simulink model "stage4"  (Simulink 7.7)
settings: Solver=ode45  StartTime=0.0  StopTime=0.1  RelTol=1e-3
undefined symbols (not defined in the file): Acid, Lead
libraries: powerlib x7, electricdrivelib x2
settings Model: Creator=Vikas  LastModifiedBy=HASANTH

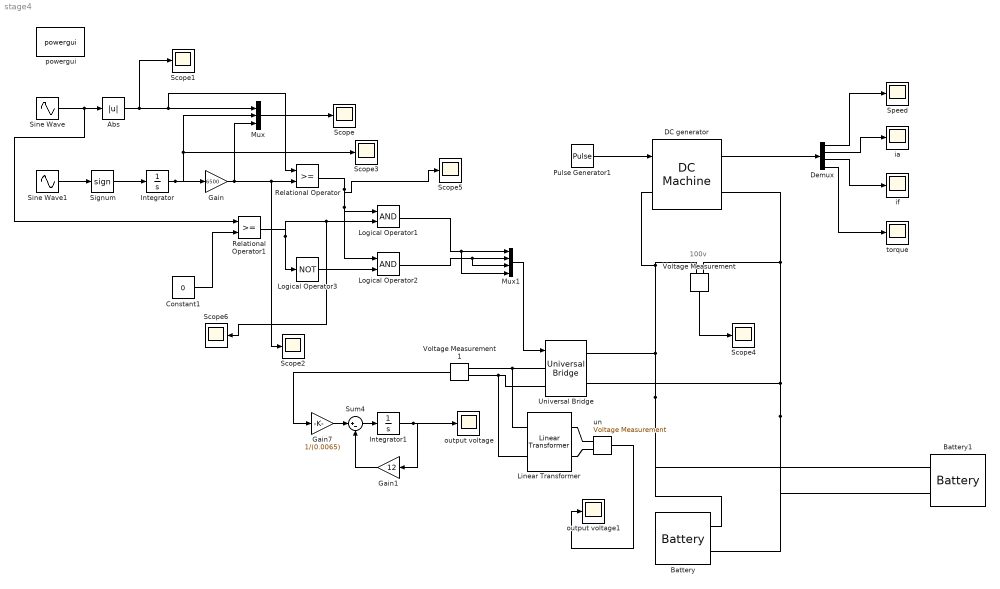
== system stage4 ==
  note: 100v
  Abs : Abs
  Battery : electricdrivelib/Extra Sources/Battery  SystemSampleTime=-1  BatType=Lead-Acid  ShowDetailedParameters=off  NomV=15  NomQ=60  SOC=20  PresetModel=on  MaxQ=62.5  FullV=16.3322  Dis_rate=12  R=0.0025  Normal_OP=18.6167  expZone="[15.2714          0.2]"  Dis_Char=off  current=[6.5 13 32.5]  Units=Time  Batt_Tr=5
  Battery1 : electricdrivelib/Extra Sources/Battery  SystemSampleTime=-1  BatType=Lead-Acid  ShowDetailedParameters=off  NomV=15  NomQ=60  SOC=20  PresetModel=on  MaxQ=62.5  FullV=16.3322  Dis_rate=12  R=0.0025  Normal_OP=18.6167  expZone="[15.2714          0.2]"  Dis_Char=off  current=[6.5 13 32.5]  Units=Time  Batt_Tr=5
  Constant1 : Constant  Value=0
  DC generator : powerlib/Machines/DC Machine  SystemSampleTime=-1  PresetModel=No  MechanicalLoad=Speed w  FieldType=Permanent magnet  ShowDetailedParameters=on  RLa="[ 1  0.012]"  RLf="[ 240  120]"  Laf=1.8  MachineConstant=Back-emf constant (V/rpm)  Ke=3  Kt=3.18  J=1  Bm=0  Tf=0  w0=1  Ifinit=1  TsPowergui=0  TsBlock=-1
      settings: AttributesFormatString=\n
  Demux : Demux
  Gain : Gain  Gain=6500
  Gain1 : Gain  Gain=12
  Gain7 : Gain  Gain=1/(0.0065)
  Integrator : Integrator
  Integrator1 : Integrator
  Linear Transformer : powerlib/Elements/Linear Transformer  PhysicalDomain=powersysdomain  SubClassName=unknown  LeftPortType=p1  RightPortType=p1  LConnTagsString=a|b  RConnTagsString=A|B  UNITS=pu  NominalPower=[ 875 50 ]  winding1="[15  0.002  0.08 ]"  winding2="[240  0.002  0.08 ]"  ThreeWindings=off  winding3=[ 315e3 0.002 0.08 ]  RmLm=[ 500 500 ]  Measurements=None  DataType=off
  Logical Operator1 : Logic  AllPortsSameDT=off  OutDataTypeStr=boolean
  Logical Operator2 : Logic  AllPortsSameDT=off  OutDataTypeStr=boolean
  Logical Operator3 : Logic  Operator=NOT  AllPortsSameDT=off  OutDataTypeStr=boolean
  Mux : Mux  Inputs=3
  Mux1 : Mux
  Pulse Generator1 : DiscretePulseGenerator  PulseType=Time based  Amplitude=5.4  Period=10  PulseWidth=50
  Relational Operator : RelationalOperator  InputSameDT=on
  Relational Operator1 : RelationalOperator  InputSameDT=on
  Scope{,1..6} (7 alike) : Scope
      Scope settings: TimeRange=10  YMin=-0.1  YMax=2.1  SaveName=ScopeData5
      Scope1 settings: TimeRange=10  YMin=-0.1  YMax=2.1  SaveName=ScopeData8
      Scope2 settings: TimeRange=10  YMin=-0.1  YMax=2.1  SaveName=ScopeData6
      Scope3 settings: TimeRange=10  YMin=-0.1  YMax=2.1  SaveName=ScopeData7
      Scope4 settings: TimeRange=1  YMin=0  YMax=36.0525  SaveName=ScopeData4
      Scope5 settings: TimeRange=10  YMin=-0.1  YMax=2.1  SaveName=ScopeData9
      Scope6 settings: TimeRange=10  YMin=-0.1  YMax=2.1  SaveName=ScopeData11
  Signum : Signum
  Sine Wave : Sin  Frequency=2*pi*50  SampleTime=0
  Sine Wave1 : Sin  Frequency=2*pi*3000  SampleTime=0
  Speed : Scope
  Sum4 : Sum  Inputs=|+-
  Universal Bridge : powerlib/Power Electronics/Universal Bridge  SystemSampleTime=-1  Arms=2  SnubberResistance=1e5  SnubberCapacitance=inf  Device=MOSFET / Diodes  Ron=1e-3  Lon=0  ForwardVoltages="[  0  0  ]"  ForwardVoltage=0  GTOparameters=[ 10e-6 , 20e-6 ]  IGBTparameters=[ 1e-6 , 2e-6 ]  Measurements=None  Measurements_2=None  converterType=Rectifier
  Voltage Measurement : powerlib/Measurements/Voltage Measurement  SystemSampleTime=-1  PhasorSimulation=off  OutputType=Complex  PSBequivalent=0
  Voltage Measurement1 : powerlib/Measurements/Voltage Measurement  SystemSampleTime=-1  PhasorSimulation=off  OutputType=Complex  PSBequivalent=0
  ia : Scope
  if : Scope
      settings: SaveName=ScopeData2
  output voltage : Scope
      settings: YMin=0.3523  YMax=0.3538  SaveName=ScopeData10
  output voltage1 : Scope
      settings: YMin=4.5e-010  YMax=7.75e-010  SaveName=ScopeData12
  powergui : powerlib/powergui  Priority=1  SystemSampleTime=-1  SimulationMode=Continuous  SampleTime=50e-6  frequency=60  SPID=off  DisableSnubberDevices=off  DisableRonSwitches=off  DisableVfSwitches=off  SwTol=0  Interpol=off  DisplayEquations=off  FunctionMessages=off  frequencyindice=0  Pbase=100e6  ErrMax=1e-4  Iterations=50  UnitsV=kV  UnitsW=MW  echomessages=off  HookPort=off  EnableUseOfTLC=off  x0status=steady  RestoreLinks=no  ResistiveCurrentMeasurement=off  Frange=[0:2:500]  Ylog=off  Xlog=on  ShowGrid=off  save=off  variable=ZData  structure=ScopeData8  ZoomFFT=off  StartTime=0.0  cycles=1  DisplayStyle=1  fundamental=60  FreqAxis=off  MaxFrequency=1000  frequencyindicesteady=1  RmsSteady=1  display=off  Ts=0  methode=off
  torque : Scope
      settings: SaveName=ScopeData3
  un : powerlib/Measurements/Voltage Measurement  SystemSampleTime=-1  PhasorSimulation=off  OutputType=Complex  PSBequivalent=0
  wires:
  DC generator/1 -> Demux/1
  Demux/1 -> Speed/1
  Demux/2 -> ia/1
  Demux/3 -> if/1
  Demux/4 -> torque/1
  Voltage Measurement/1 -> Scope4/1
  Pulse Generator1/1 -> DC generator/1
  Sine Wave/1 -> Abs/1, Relational Operator1/1
  Abs/1 -> Mux/1, Relational Operator/1, Scope1/1
  Mux/1 -> Scope/1
  Sine Wave1/1 -> Signum/1
  Signum/1 -> Integrator/1
  Integrator/1 -> Gain/1, Mux/2, Scope3/1
  Gain/1 -> Relational Operator/2, Scope2/1, Mux/3
  Logical Operator3/1 -> Logical Operator2/2
  Relational Operator/1 -> Logical Operator1/1, Logical Operator2/1, Scope5/1
  Constant1/1 -> Relational Operator1/2
  Relational Operator1/1 -> Logical Operator3/1, Logical Operator1/2, Scope6/1
  Mux1/1 -> Universal Bridge/1
  Logical Operator1/1 -> Mux1/1, Mux1/4
  Logical Operator2/1 -> Mux1/2, Mux1/3
  Integrator1/1 -> Gain1/1, output voltage/1
  Gain7/1 -> Sum4/1
  Sum4/1 -> Integrator1/1
  Gain1/1 -> Sum4/2
  Voltage Measurement1/1 -> Gain7/1
  un/1 -> output voltage1/1
  connections:
  Universal Bridge/LConn1 -- Voltage Measurement1/LConn1 -- Linear Transformer/LConn1
  Universal Bridge/LConn2 -- Voltage Measurement1/LConn2 -- Linear Transformer/LConn2
  Battery/LConn1 -- Battery1/LConn1 -- Universal Bridge/RConn1 -- DC generator/LConn1 -- Voltage Measurement/LConn1
  DC generator/RConn1 -- Battery/LConn2 -- Battery1/LConn2 -- Universal Bridge/RConn2 -- Voltage Measurement/LConn2
  un/LConn1 -- Linear Transformer/RConn1
  un/LConn2 -- Linear Transformer/RConn2
